simulink model "SG_direct_DLE_position_control_hose_pump"  (R2025b)
settings: Solver=FixedStepAuto  StartTime=0.0  StopTime=inf  FixedStep=0.0001  RelTol=1e-3
libraries: simulink x3, SG_DLE_position_control_module_hose_pump x1, servo_valve_pressure_control_module x1
settings Model: Creator=cmmcguir  LastModifiedBy=cmmcguir
settings SolverCC: ConcurrentTasks=on  PositivePriorityOrder=on
settings OptimizationCC: BlockReduction=off  OptimizeBlockIOStorage=off
settings DebuggingCC: TasksWithSamePriorityMsg=none
settings HardwareCC: ProdBitPerLong=64.0  ProdLongLongMode=on  ProdHWDeviceType=Intel->x86-64 (Linux 64)
settings RTWCC: SystemTargetFile=speedgoat.tlc  TemplateMakefile=slrealtime_default_tmf  Toolchain=Simulink Real-Time Toolchain  BuildConfiguration=Faster Runs  CodeExecutionProfiling=on  TargetLang=C++  Description=Speedgoat Real-Time Target Machine
settings SimulinkRealTimeTargetCC: SLRTFileLogMaxRuns=1.0  ExtModeMaxTrigDuration=10.0  ExtModeStaticAllocSize=1000000.0  ExtModeTransport=0.0  MultiwordLength=2048.0  DynamicStringBufferSize=256.0  PreserveMATLABNamespacesInGeneratedCode=on  SubcomponentCodeInterfacePackaging=Reusable function  MATLABClassNameForMDSCustomization=Simulink.SoftwareTarget.GRTCustomization  InstructionSetFMA=off  LogToMDFFile=off

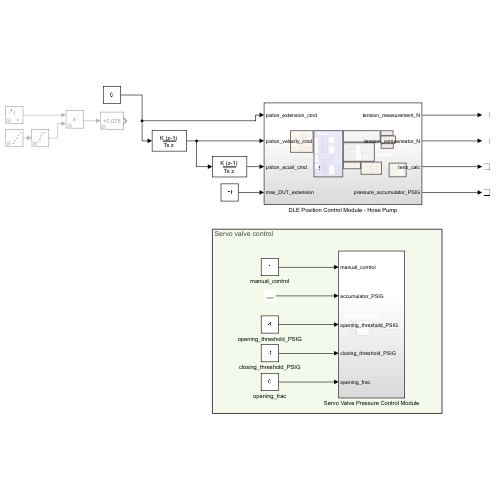
[thumbnail: Simulink's stored preview of the top-level diagram]
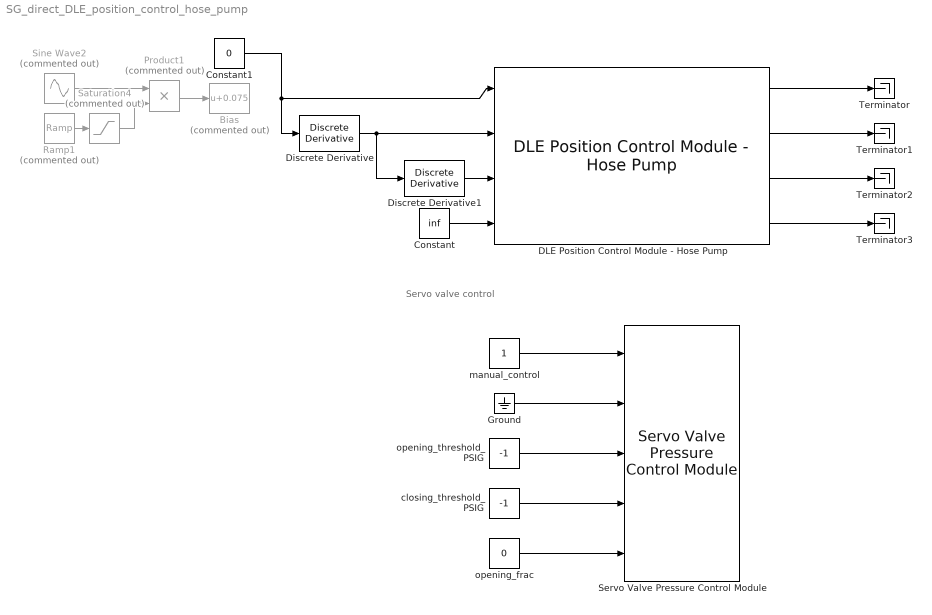
== system SG_direct_DLE_position_control_hose_pump ==
  note: Servo valve control
  Bias : Bias  Commented=on  Bias=0.075  SaturateOnIntegerOverflow=off
  Constant : Constant  Value=inf
  Constant1 : Constant  Value=0
  DLE Position Control Module - Hose Pump : SG_DLE_position_control_module_hose_pump/DLE Position Control Module - Hose Pump  SystemSampleTime=-1  VariantActivationTime=update diagram  EmptyChoice=off  PassThrough=off  PassThroughVariantControl=(default)  EmptyChoiceVariantControl=(default)  AllowFlexibleInterface=on  Latency=0  AutoFrameSizeCalculation=off
  Discrete Derivative : simulink/Discrete/Discrete Derivative  gainval=1.0  ICPrevScaledInput=0.0  OutMin=[]  OutMax=[]  OutDataType=fixdt(1, 16)  OutScaling=2^-10  DoSatur=off
  Discrete Derivative1 : simulink/Discrete/Discrete Derivative  gainval=1.0  ICPrevScaledInput=0.0  OutMin=[]  OutMax=[]  OutDataType=fixdt(1, 16)  OutScaling=2^-10  DoSatur=off
  Ground : Ground
  Product1 : Product  Commented=on
  Ramp1 : simulink/Sources/Ramp  Commented=on  slope=1/10  start=10  InitialOutput=0
  Saturation4 : Saturate  Commented=on  UpperLimit=1  LowerLimit=0
  Servo Valve Pressure Control Module : servo_valve_pressure_control_module/Servo Valve Pressure Control Module  SystemSampleTime=-1  VariantActivationTime=update diagram  EmptyChoice=off  PassThrough=off  PassThroughVariantControl=(default)  EmptyChoiceVariantControl=(default)  AllowFlexibleInterface=on  Latency=0  AutoFrameSizeCalculation=off
  Sine Wave2 : Sin  Commented=on  Amplitude=0.03  Frequency=2*pi/1.75  SampleTime=0.0001
  Terminator{,1..3} (4 alike) : Terminator
  closing_threshold_PSIG : Constant  Value=-1
  manual_control : Constant  SampleTime=0.0001
  opening_frac : Constant  Value=0
  opening_threshold_PSIG : Constant  Value=-1
  wires:
  Saturation4/1 -> Product1/2
  Ramp1/1 -> Saturation4/1
  Sine Wave2/1 -> Product1/1
  Product1/1 -> Bias/1
  Discrete Derivative/1 -> Discrete Derivative1/1, DLE Position Control Module - Hose Pump/2
  Discrete Derivative1/1 -> DLE Position Control Module - Hose Pump/3
  DLE Position Control Module - Hose Pump/1 -> Terminator/1
  DLE Position Control Module - Hose Pump/2 -> Terminator1/1
  Constant1/1 -> DLE Position Control Module - Hose Pump/1, Discrete Derivative/1
  Ground/1 -> Servo Valve Pressure Control Module/2
  closing_threshold_PSIG/1 -> Servo Valve Pressure Control Module/4
  opening_frac/1 -> Servo Valve Pressure Control Module/5
  manual_control/1 -> Servo Valve Pressure Control Module/1
  opening_threshold_PSIG/1 -> Servo Valve Pressure Control Module/3
  DLE Position Control Module - Hose Pump/4 -> Terminator3/1
  DLE Position Control Module - Hose Pump/3 -> Terminator2/1
  Constant/1 -> DLE Position Control Module - Hose Pump/4
